simulink model "rotorparameters"  (Simulink 7.3)
settings: Solver=ode23t  StartTime=0.0  StopTime=0.9  RelTol=1e-3
libraries: powerlib x1
settings Model: Creator=lenovo  LastModifiedBy=lenovo

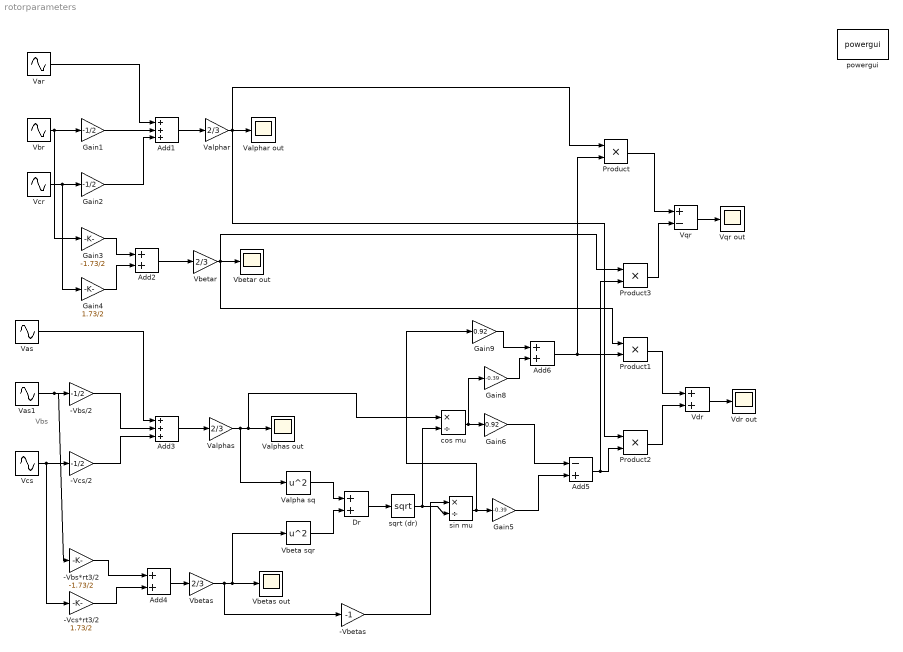
== system rotorparameters ==
  note: Vbs
  "-Vbetas " : Gain  Gain=-1  ParameterDataType=fixdt(1, 16)  ParameterScaling=2^0  OutDataType=fixdt(1, 16)  OutScaling=2^0
  -Vbs*rt3/2 : Gain  Gain=-1.73/2  ParameterDataType=fixdt(1, 16)  ParameterScaling=2^0  OutDataType=fixdt(1, 16)  OutScaling=2^0
  -Vbs/2 : Gain  Gain=-1/2  ParameterDataType=fixdt(1, 16)  ParameterScaling=2^0  OutDataType=fixdt(1, 16)  OutScaling=2^0
  -Vcs*rt3/2 : Gain  Gain=1.73/2  ParameterDataType=fixdt(1, 16)  ParameterScaling=2^0  OutDataType=fixdt(1, 16)  OutScaling=2^0
  -Vcs/2 : Gain  Gain=-1/2  ParameterDataType=fixdt(1, 16)  ParameterScaling=2^0  OutDataType=fixdt(1, 16)  OutScaling=2^0
  Add1 : Sum  Inputs=+++  OutDataType=fixdt(1, 16)  OutScaling=2^-10
  Add2 : Sum  OutDataType=fixdt(1, 16)  OutScaling=2^-10
  Add3 : Sum  Inputs=+++  OutDataType=fixdt(1, 16)  OutScaling=2^-10
  Add4 : Sum  OutDataType=fixdt(1, 16)  OutScaling=2^-10
  Add5 : Sum  Inputs=-+  OutDataType=fixdt(1, 16)  OutScaling=2^-10
  Add6 : Sum  OutDataType=fixdt(1, 16)  OutScaling=2^-10
  Dr : Sum  OutDataType=fixdt(1, 16)  OutScaling=2^-10
  Gain1 : Gain  Gain=-1/2  ParameterDataType=fixdt(1, 16)  ParameterScaling=2^0  OutDataType=fixdt(1, 16)  OutScaling=2^0
  Gain2 : Gain  Gain=-1/2  ParameterDataType=fixdt(1, 16)  ParameterScaling=2^0  OutDataType=fixdt(1, 16)  OutScaling=2^0
  Gain3 : Gain  Gain=-1.73/2  ParameterDataType=fixdt(1, 16)  ParameterScaling=2^0  OutDataType=fixdt(1, 16)  OutScaling=2^0
  Gain4 : Gain  Gain=1.73/2  ParameterDataType=fixdt(1, 16)  ParameterScaling=2^0  OutDataType=fixdt(1, 16)  OutScaling=2^0
  Gain5 : Gain  Gain=-0.39  ParameterDataType=fixdt(1, 16)  ParameterScaling=2^0  OutDataType=fixdt(1, 16)  OutScaling=2^0
  Gain6 : Gain  Gain=0.92  ParameterDataType=fixdt(1, 16)  ParameterScaling=2^0  OutDataType=fixdt(1, 16)  OutScaling=2^0
  Gain8 : Gain  Gain=-0.39  ParameterDataType=fixdt(1, 16)  ParameterScaling=2^0  OutDataType=fixdt(1, 16)  OutScaling=2^0
  Gain9 : Gain  Gain=0.92  ParameterDataType=fixdt(1, 16)  ParameterScaling=2^0  OutDataType=fixdt(1, 16)  OutScaling=2^0
  Product{,1..3} (4 alike) : Product  OutDataType=fixdt(1, 16)  OutScaling=2^0  RndMeth=Zero
  Valpha sq : Math  Operator=square  OutDataType=fixdt(1, 16)  OutScaling=2^0  SaturateOnIntegerOverflow=on
  Valphar : Gain  Gain=2/3  ParameterDataType=fixdt(1, 16)  ParameterScaling=2^0  OutDataType=fixdt(1, 16)  OutScaling=2^0
  Valphar out : Scope
      settings: YMin=-300  YMax=300
  Valphas : Gain  Gain=2/3  ParameterDataType=fixdt(1, 16)  ParameterScaling=2^0  OutDataType=fixdt(1, 16)  OutScaling=2^0
  Valphas out : Scope
      settings: YMin=-300  YMax=300  SaveName=ScopeData4
  Var : Sin  Amplitude=230  Bias=0  Frequency=314  Phase=0  Samples=10  SampleTime=0  Offset=0
  Vas : Sin  Amplitude=230  Bias=0  Frequency=314  Phase=0  Samples=10  SampleTime=0  Offset=0
  Vas1 : Sin  Amplitude=230  Bias=0  Frequency=314  Phase=-2.09  Samples=10  SampleTime=0  Offset=0
  Vbeta sqr : Math  Operator=square  OutDataType=fixdt(1, 16)  OutScaling=2^0  SaturateOnIntegerOverflow=on
  Vbetar : Gain  Gain=2/3  ParameterDataType=fixdt(1, 16)  ParameterScaling=2^0  OutDataType=fixdt(1, 16)  OutScaling=2^0
  Vbetar out : Scope
      settings: YMin=-300  YMax=300  SaveName=ScopeData2
  Vbetas : Gain  Gain=2/3  ParameterDataType=fixdt(1, 16)  ParameterScaling=2^0  OutDataType=fixdt(1, 16)  OutScaling=2^0
  Vbetas out : Scope
      settings: YMin=-300  YMax=300  SaveName=ScopeData5
  Vbr : Sin  Amplitude=230  Bias=0  Frequency=314  Phase=-2.09  Samples=10  SampleTime=0  Offset=0
  Vcr : Sin  Amplitude=230  Bias=0  Frequency=314  Phase=-4.18  Samples=10  SampleTime=0  Offset=0
  Vcs : Sin  Amplitude=230  Bias=0  Frequency=314  Phase=-4.18  Samples=10  SampleTime=0  Offset=0
  Vdr : Sum  OutDataType=fixdt(1, 16)  OutScaling=2^-10
  Vdr out : Scope
      settings: YMin=-300  YMax=300  SaveName=ScopeData3
  Vqr : Sum  Inputs=+-  OutDataType=fixdt(1, 16)  OutScaling=2^-10
  Vqr out : Scope
      settings: YMin=-300  YMax=300  SaveName=ScopeData6
  cos mu : Product  Inputs=*/  OutDataType=fixdt(1, 16)  OutScaling=2^-10
  powergui : powerlib/powergui  Priority=1  SystemSampleTime=-1  SimulationMode=Continuous  SampleTime=50e-6  frequency=60  SPID=off  DisableSnubberDevices=off  DisableRonSwitches=off  DisableVfSwitches=off  SwTol=0  Interpol=off  frequencyindice=60  echomessages=off  HookPort=off  DisplayEquations=off  FunctionMessages=off  EnableUseOfTLC=off  x0status=blocks  RestoreLinks=warning  Frange=[0:2:500]  Ylog=off  Xlog=on  ShowGrid=off  save=off  variable=ZData  ZoomFFT=on  StartTime=0.0  cycles=1  DisplayStyle=1  fundamental=60  FreqAxis=off  MaxFrequency=1000  frequencyindicesteady=1  RmsSteady=1  display=off  Ts=0  methode=off
  sin mu : Product  Inputs=*/  OutDataType=fixdt(1, 16)  OutScaling=2^-10
  sqrt (dr) : Math  Operator=sqrt  OutDataType=fixdt(1, 16)  OutScaling=2^0  SaturateOnIntegerOverflow=on
  wires:
  Vbr/1 -> Gain1/1, Gain3/1
  Vcr/1 -> Gain2/1, Gain4/1
  Gain1/1 -> Add1/2
  Gain2/1 -> Add1/3
  Var/1 -> Add1/1
  Add1/1 -> Valphar/1
  Valphar/1 -> Valphar out/1, Product2/1, Product/1
  Gain3/1 -> Add2/1
  Gain4/1 -> Add2/2
  Add2/1 -> Vbetar/1
  Vbetar/1 -> Vbetar out/1, Product1/1, Product3/1
  Vas1/1 -> -Vbs/2/1, -Vbs*rt3/2/1
  Vcs/1 -> -Vcs/2/1, -Vcs*rt3/2/1
  Vas/1 -> Add3/1
  -Vbs/2/1 -> Add3/2
  -Vcs/2/1 -> Add3/3
  Add3/1 -> Valphas/1
  -Vbs*rt3/2/1 -> Add4/1
  Add4/1 -> Vbetas/1
  Valphas/1 -> Valpha sq/1, Valphas out/1, cos mu/1
  Vbetas/1 -> Vbeta sqr/1, Vbetas out/1, "-Vbetas "/1
  Valpha sq/1 -> Dr/1
  Vbeta sqr/1 -> Dr/2
  Dr/1 -> sqrt (dr)/1
  "-Vbetas "/1 -> sin mu/1
  sqrt (dr)/1 -> sin mu/2, cos mu/2
  sin mu/1 -> Gain5/1, Gain9/1
  cos mu/1 -> Gain6/1, Gain8/1
  Gain6/1 -> Add5/1
  Gain5/1 -> Add5/2
  Add5/1 -> Product2/2, Product3/2
  Gain9/1 -> Add6/1
  Gain8/1 -> Add6/2
  Add6/1 -> Product1/2, Product/2
  Product1/1 -> Vdr/1
  Product2/1 -> Vdr/2
  Vdr/1 -> Vdr out/1
  Product/1 -> Vqr/1
  Product3/1 -> Vqr/2
  Vqr/1 -> Vqr out/1
  -Vcs*rt3/2/1 -> Add4/2
